simulink model "SIM_6DOF"  (R2021b)
settings: Solver=FixedStepAuto  StartTime=0.0  StopTime=D.Tfim  FixedStep=0.001  MaxStep=0.001  RelTol=1e-3
undefined symbols (not defined in the file or in its folder): c, D, dados, desv_emp, erro, F, Light, M, MIL, Newton, Raphson, wind
libraries: aerolibasang x7, sharedutil x3, aerolibwind2 x3, shared6dof x2, aerolibanim x1, aerolibatmos2 x1, simulink x1, dspmtrx3 x1, sharedtransform x1
settings Model: Creator=carlberto-old  LastModifiedBy=user
settings SolverCC: AlgebraicLoopSolver=LineSearch
settings DataIOCC: SaveFormat=Array  ReturnWorkspaceOutputs=off
settings DebuggingCC: SFMachineParentedDataDiag=warning  ArithmeticOperatorsInVariantConditions=warning
settings SFSimCC: SimUseLocalCustomCode=off  CustomCodeUndefinedFunction=UseInterfaceOnly
settings RTWCC: RTWUseLocalCustomCode=off

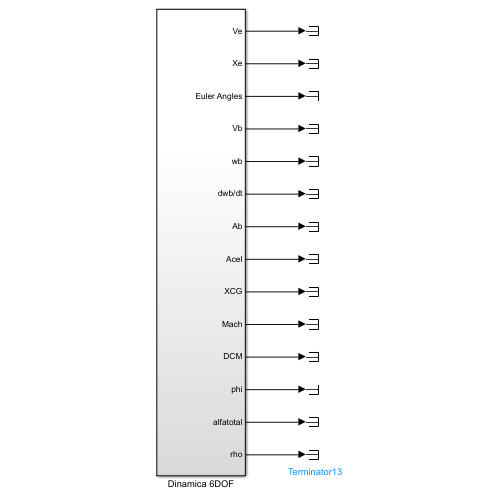
[thumbnail: Simulink's stored preview of the top-level diagram]
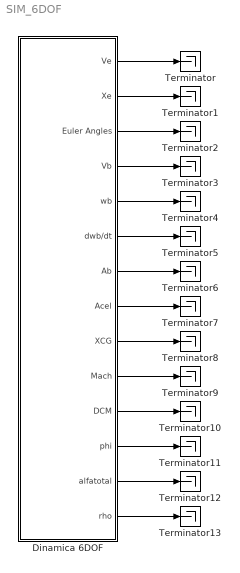
== system SIM_6DOF ==
  Dinamica 6DOF : Subsystem
  Terminator{,1..13} (14 alike) : Terminator
  wires:
  Dinamica 6DOF/3(Euler Angles) -> Terminator2/1
  Dinamica 6DOF/5(wb) -> Terminator4/1
  Dinamica 6DOF/1(Ve) -> Terminator/1
  Dinamica 6DOF/7(Ab) -> Terminator6/1
  Dinamica 6DOF/6(dwb/dt) -> Terminator5/1
  Dinamica 6DOF/11(DCM) -> Terminator10/1
  Dinamica 6DOF/9(XCG) -> Terminator8/1
  Dinamica 6DOF/8(Acel) -> Terminator7/1
  Dinamica 6DOF/10(Mach) -> Terminator9/1
  Dinamica 6DOF/12(phi) -> Terminator11/1
  Dinamica 6DOF/13(alfatotal) -> Terminator12/1
  Dinamica 6DOF/14(rho) -> Terminator13/1
  Dinamica 6DOF/2(Xe) -> Terminator1/1
  Dinamica 6DOF/4(Vb) -> Terminator3/1

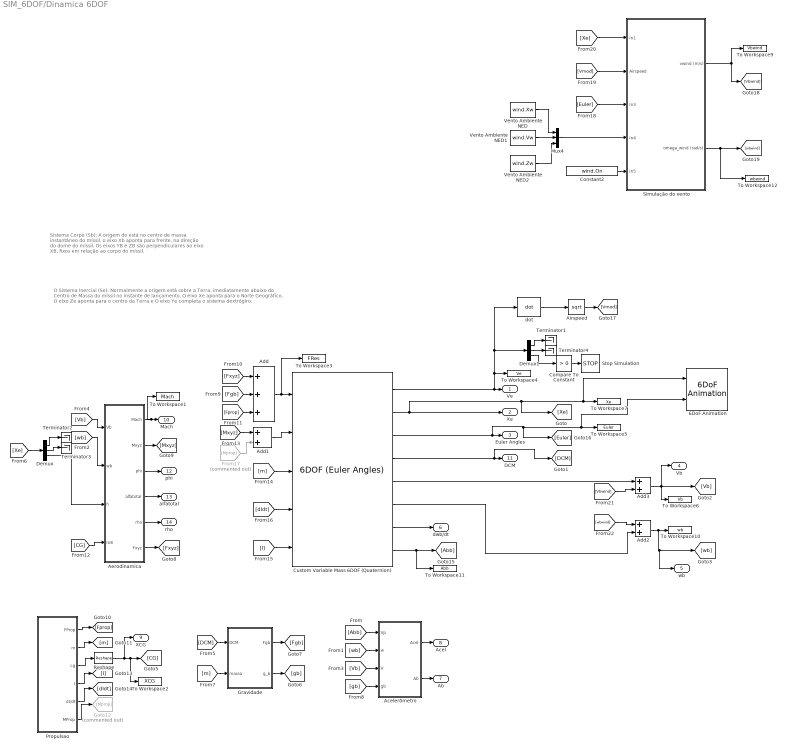
== system SIM_6DOF/Dinamica 6DOF ==
  note: O Sistema Inercial (Se):
      | Normalmente a origem está sobre a Terra, imediatamente abaixo do Centro de Massa do míssil no instante de lançamento.
      | O eixo Xe aponta para o Norte Geográfico,
      | O eixo Ze aponta para o centro da Terra e
      | O eixo Ye completa o sistema dextrógiro.
  note: Sistema Corpo (Sb):
      | A origem do está no centro de massa instantâneo do míssil.
      | o eixo Xb aponta para frente, na direção do dome do míssil.
      | Os eixos YB e ZB são perpendiculares ao eixo XB, fixos
      | em relação ao corpo do míssil.
  6DoF Animation : aerolibanim/6DoF Animation  u1=[0 4000 -2000 2000 -1000 6000]  u2=0.1  u3=1  u4=[0 0 0]  u5=Fly alongside  u6=[0 30 0]  u7=10  u8=on
  Acelerômetro : Subsystem
  Add : Sum  Inputs=+++
  Add1 : Sum
  Add2 : Sum
  Add3 : Sum
  Aerodinamica : Subsystem
  Airspeed : Sqrt  AlgorithmType=Newton-Raphson  SaturateOnIntegerOverflow=on
  Compare To Constant : simulink/Logic and Bit Operations/Compare To Constant  relop=>  const=0  OutDataTypeStr=boolean
  Constant2 : Constant  Value=wind.On
  Custom Variable Mass 6DOF (Quaternion) : shared6dof/6DOF (Euler Angles)  units=Metric (MKS)  mtype=Custom Variable  rep=Quaternion  xme_0=[0 0 -D.Alt0]  Vm_0=[D.U 0 0]  eul_0="[D.phi0  D.theta0   D.psi0]"  pm_0=[D.p0 D.q0 D.r0]  mass_0=1.0  mass_e=0.5  mass_f=2.0  inertia=eye(3)  inertia_e=eye(3)  inertia_f=2*eye(3)  k_quat=D.Kq  vre_flag=off  abi_flag=off  aMode=aMode  xme_statename=''  Vm_statename=''  eul_statename=''  quat_statename=''  pm_statename=''  mass_statename=''
      settings: SourceProductBaseCode=AE,PW,DR,MT,UV,VE
  Demux : Demux  Outputs=3
  Demux1 : Demux  Outputs=3
  From17 : From  Commented=on  GotoTag=Mprop
  Goto12 : Goto  Commented=on  GotoTag=Mprop
  Gravidade : Subsystem
  Mux4 : Mux  Inputs=3
  Propulsao : Subsystem
  Reshape : Reshape
  Simulação do vento : Subsystem
  Stop Simulation : Stop
  Terminator{1..4} (4 alike) : Terminator
  To Workspace1 : ToWorkspace  VariableName=Mach  SaveFormat=Timeseries  SampleTime=-1
  To Workspace10 : ToWorkspace  VariableName=wb  SaveFormat=Timeseries  SampleTime=-1
  To Workspace11 : ToWorkspace  VariableName=Abb  SaveFormat=Timeseries  SampleTime=-1
  To Workspace12 : ToWorkspace  VariableName=wbwind  SaveFormat=Timeseries  SampleTime=-1
  To Workspace2 : ToWorkspace  VariableName=XCG  SaveFormat=Timeseries  SampleTime=-1
  To Workspace3 : ToWorkspace  VariableName=FRes  SaveFormat=Timeseries  SampleTime=-1
  To Workspace4 : ToWorkspace  VariableName=Ve  SaveFormat=Timeseries  SampleTime=-1
  To Workspace5 : ToWorkspace  VariableName=Euler  SaveFormat=Timeseries  SampleTime=-1
  To Workspace6 : ToWorkspace  VariableName=Vb  SaveFormat=Timeseries  SampleTime=-1
  To Workspace7 : ToWorkspace  VariableName=Xe  SaveFormat=Timeseries  SampleTime=-1
  To Workspace9 : ToWorkspace  VariableName=Vbwind  SaveFormat=Timeseries  SampleTime=-1
  Vento Ambiente NED : Constant  Value=wind.Xw
  Vento Ambiente NED1 : Constant  Value=wind.Vw
  Vento Ambiente NED2 : Constant  Value=wind.Zw
  dot : aerolibasang/Incidence, Sideslip, & Airspeed/dot  SystemSampleTime=-1  VariantActivationTime=update diagram  Latency=0  AutoFrameSizeCalculation=off
      settings: SourceProductBaseCode=AE
  Ve : Outport  VectorParamsAs1DForOutWhenUnconnected=off
  Xe : Outport  Port=2  VectorParamsAs1DForOutWhenUnconnected=off
  Euler Angles : Outport  Port=3  VectorParamsAs1DForOutWhenUnconnected=off
  Vb : Outport  Port=4  VectorParamsAs1DForOutWhenUnconnected=off
  wb : Outport  Port=5  VectorParamsAs1DForOutWhenUnconnected=off
  dwb/dt : Outport  Port=6  VectorParamsAs1DForOutWhenUnconnected=off
  Ab : Outport  Port=7  VectorParamsAs1DForOutWhenUnconnected=off
  Acel : Outport  Port=8  VectorParamsAs1DForOutWhenUnconnected=off
  XCG : Outport  Port=9  VectorParamsAs1DForOutWhenUnconnected=off
  Mach : Outport  Port=10  VectorParamsAs1DForOutWhenUnconnected=off
  DCM : Outport  Port=11  VectorParamsAs1DForOutWhenUnconnected=off
  phi : Outport  Port=12  VectorParamsAs1DForOutWhenUnconnected=off
  alfatotal : Outport  Port=13  VectorParamsAs1DForOutWhenUnconnected=off
  rho : Outport  Port=14  VectorParamsAs1DForOutWhenUnconnected=off
  wires:
  Custom Variable Mass 6DOF (Quaternion)/1 -> To Workspace4/1, dot/1, Demux1/1, Ve/1
  Custom Variable Mass 6DOF (Quaternion)/7 -> dwb/dt/1
  Demux/1 -> Terminator2/1
  Demux/2 -> Terminator3/1
  Add/1 -> To Workspace3/1, Custom Variable Mass 6DOF (Quaternion)/1
  Custom Variable Mass 6DOF (Quaternion)/4 -> [DCM], DCM/1
  Demux/3 -> Aerodinamica/3(h)
  Aerodinamica/1(Mach) -> To Workspace1/1, Mach/1
  Propulsao/3(cg) -> Reshape/1
  [Abb] -> Acelerômetro/1(Vp)
  [wb] -> Acelerômetro/2(w)
  [wb] -> Aerodinamica/2(wb)
  [Vb] -> Acelerômetro/3(V)
  [Vb] -> Aerodinamica/1(Vb)
  [DCM] -> Gravidade/1(DCM)
  [Xe] -> Demux/1
  Acelerômetro/2(Ab) -> Ab/1
  [gb] -> Acelerômetro/4(gb)
  Aerodinamica/6(" Fxyz") -> [Fxyz]
  Aerodinamica/2(Mxyz) -> [Mxyz]
  Propulsao/1(FProp) -> [Fprop]
  Propulsao/2(m) -> [m]
  Propulsao/4(I) -> [I]
  Propulsao/5(dI/dt) -> [dIdt]
  [m] -> Custom Variable Mass 6DOF (Quaternion)/3
  [I] -> Custom Variable Mass 6DOF (Quaternion)/5
  [dIdt] -> Custom Variable Mass 6DOF (Quaternion)/4
  Custom Variable Mass 6DOF (Quaternion)/8 -> [Abb], To Workspace11/1
  Aerodinamica/3(phi) -> phi/1
  Aerodinamica/4(alfatotal) -> alfatotal/1
  Aerodinamica/5(rho) -> rho/1
  [m] -> Gravidade/2(massa)
  Gravidade/1(Fgb) -> [Fgb]
  Acelerômetro/1(Acel) -> Acel/1
  Gravidade/2(g_b) -> [gb]
  [Fprop] -> Add/3
  Add1/1 -> Custom Variable Mass 6DOF (Quaternion)/2
  Propulsao/6(MProp) -> Goto12/1
  Demux1/3 -> Compare To Constant/1
  Demux1/2 -> Terminator4/1
  Demux1/1 -> Terminator1/1
  Compare To Constant/1 -> Stop Simulation/1
  From17/1 -> Add1/2
  [Mxyz] -> Add1/1
  [Fgb] -> Add/2
  [Fxyz] -> Add/1
  [CG] -> Aerodinamica/4(In8)
  Custom Variable Mass 6DOF (Quaternion)/3 -> [Euler], 6DoF Animation/2, To Workspace5/1, Euler Angles/1
  Add3/1 -> Vb/1, To Workspace6/1, [Vb]
  Add2/1 -> wb/1, [wb], To Workspace10/1
  Custom Variable Mass 6DOF (Quaternion)/6 -> Add2/2
  Custom Variable Mass 6DOF (Quaternion)/5 -> Add3/1
  [Vbwind] -> Add3/2
  [wbwind] -> Add2/1
  Vento Ambiente NED2/1 -> Mux4/3
  Vento Ambiente NED1/1 -> Mux4/2
  Vento Ambiente NED/1 -> Mux4/1
  dot/1 -> Airspeed/1
  Airspeed/1 -> [Vmod]
  Custom Variable Mass 6DOF (Quaternion)/2 -> [Xe], 6DoF Animation/1, To Workspace7/1, Xe/1
  Reshape/1 -> XCG/1, To Workspace2/1, [CG]
  Simulação do vento/2(omega_wind (rad/s)) -> To Workspace12/1, [wbwind]
  Simulação do vento/1(vwind (m/s)) -> To Workspace9/1, [Vbwind]
  [Xe] -> Simulação do vento/1(In1)
  [Vmod] -> Simulação do vento/2(Airspeed)
  [Euler] -> Simulação do vento/3(In3)
  Mux4/1 -> Simulação do vento/4(In4)
  Constant2/1 -> Simulação do vento/5(In5)

== system SIM_6DOF/Dinamica 6DOF/Acelerômetro ==
  Vp : Inport
  w : Inport  Port=2
  V : Inport  Port=3
  gb : Inport  Port=4
  Add1 : Sum
  Add2 : Sum  Inputs=+-
  To Workspace4 : ToWorkspace  VariableName=Acel  SaveFormat=Timeseries  SampleTime=-1
  To Workspace5 : ToWorkspace  VariableName=Ab  SaveFormat=Timeseries  SampleTime=-1
  w x V : sharedutil/3x3 Cross Product  aMode=aMode
      settings: SourceProductBaseCode=AE,PW,DR,MT,UV,VE
  Acel : Outport  VectorParamsAs1DForOutWhenUnconnected=off
  Ab : Outport  Port=2  VectorParamsAs1DForOutWhenUnconnected=off
  wires:
  V/1 -> w x V/2
  w/1 -> w x V/1
  Add1/1 -> Add2/1, Ab/1, To Workspace5/1
  Add2/1 -> To Workspace4/1, Acel/1
  gb/1 -> Add2/2
  w x V/1 -> Add1/2
  Vp/1 -> Add1/1

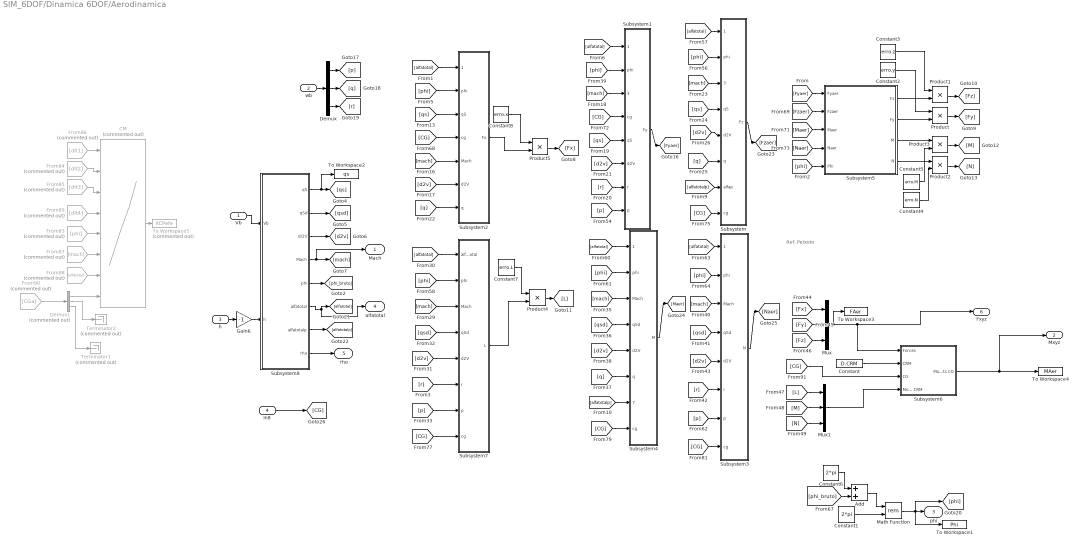
== system SIM_6DOF/Dinamica 6DOF/Aerodinamica ==
  note: Ref. Peixoto
  Vb : Inport
  wb : Inport  Port=2
  h : Inport  Port=3
  In8 : Inport  Port=4
  Add : Sum
  CM : Lookup_n-D  Commented=on  NumberOfTableDimensions=8  BreakpointsForDimension1=dados.delta1  BreakpointsForDimension2=dados.delta2  BreakpointsForDimension3=dados.delta3  BreakpointsForDimension4=dados.delta4  BreakpointsForDimension5=dados.phif  BreakpointsForDimension6=dados.mach  BreakpointsForDimension7=dados.alpha  BreakpointsForDimension8=dados.cg  Table=M.XCP  ExtrapMethod=Clip  InternalRulePriority=Speed  RndMeth=Simplest  InputSameDT=on
      settings: InputPortMap=u0,u1,u2,u3,u4,u5,u6,u7
  Constant : Constant  Value=D.CRM
  Constant1 : Constant  Value=2*pi
  Constant2 : Constant  Value=erro.y
  Constant3 : Constant  Value=erro.z
  Constant4 : Constant  Value=erro.N
  Constant5 : Constant  Value=erro.M
  Constant6 : Constant  Value=2*pi
  Constant7 : Constant  Value=erro.L
  Constant8 : Constant  Value=erro.x
  Demux : Demux  Outputs=3
  Demux1 : Demux  Commented=on  Outputs=3
  From83 : From  Commented=on  GotoTag=phi
  From84 : From  Commented=on  GotoTag=dlt2
  From85 : From  Commented=on  GotoTag=dlt3
  From86 : From  Commented=on  GotoTag=dlt1
  From87 : From  Commented=on  GotoTag=mach
  From88 : From  Commented=on  GotoTag=alfatotal
  From89 : From  Commented=on  GotoTag=dlt4
  From90 : From  Commented=on  GotoTag=CGa
  Gain6 : Gain  Gain=-1
  Math Function : Math  Operator=rem  SignedPower=on  SaturateOnIntegerOverflow=on
  Mux : Mux  Inputs=3
  Mux1 : Mux  Inputs=3
  Product{,1..5} (6 alike) : Product
  Subsystem : Subsystem
  Subsystem1 : Subsystem
  Subsystem2 : Subsystem
  Subsystem3 : Subsystem
  Subsystem4 : Subsystem
  Subsystem5 : Subsystem
  Subsystem6 : Subsystem
  Subsystem7 : Subsystem
  Subsystem8 : Subsystem
  Terminator1 : Terminator  Commented=on
  Terminator2 : Terminator  Commented=on
  To Workspace1 : ToWorkspace  VariableName=Phi  SaveFormat=Timeseries  SampleTime=-1
  To Workspace2 : ToWorkspace  VariableName=qs  SaveFormat=Timeseries  SampleTime=-1
  To Workspace3 : ToWorkspace  VariableName=FAer  SaveFormat=Timeseries  SampleTime=-1
  To Workspace4 : ToWorkspace  VariableName=MAer  SaveFormat=Timeseries  SampleTime=-1
  To Workspace5 : ToWorkspace  Commented=on  VariableName=XCPefe  SaveFormat=Timeseries  SampleTime=-1
  Mach : Outport  VectorParamsAs1DForOutWhenUnconnected=off
  Mxyz : Outport  Port=2  VectorParamsAs1DForOutWhenUnconnected=off
  phi : Outport  Port=3  VectorParamsAs1DForOutWhenUnconnected=off
  alfatotal : Outport  Port=4  VectorParamsAs1DForOutWhenUnconnected=off
  rho : Outport  Port=5  VectorParamsAs1DForOutWhenUnconnected=off
  " Fxyz" : Outport  Port=6  VectorParamsAs1DForOutWhenUnconnected=off
  wires:
  h/1 -> Gain6/1
  Mux/1 -> To Workspace3/1, Subsystem6/1(Forces), " Fxyz"/1
  wb/1 -> Demux/1
  Vb/1 -> Subsystem8/1(Vb)
  Gain6/1 -> Subsystem8/2(h)
  Constant/1 -> Subsystem6/2(CRM)
  [alfatotal] -> Subsystem2/1(alfatotal)
  [phi] -> Subsystem2/2(phi)
  [alfatotalp] -> Subsystem4/7(alfaponto)
  Subsystem8/1(qS) -> To Workspace2/1, [qs]
  Subsystem8/2(qSd) -> [qsd]
  Subsystem8/3(d/2V) -> [d2v]
  Subsystem8/4(Mach) -> Mach/1, [mach]
  [qs] -> Subsystem2/3(qS)
  [mach] -> Subsystem2/5("Mach ")
  [mach] -> Subsystem1/3("Mach ")
  [d2v] -> Subsystem7/5(d2V)
  [qsd] -> Subsystem7/4(qSd)
  [p] -> Subsystem7/7(p)
  [mach] -> Subsystem4/3("Mach ")
  [qsd] -> Subsystem4/4(qSd)
  [q] -> Subsystem4/6(q)
  [d2v] -> Subsystem4/5(d2V)
  [mach] -> Subsystem3/3("Mach ")
  [qsd] -> Subsystem3/4(qSd)
  [r] -> Subsystem3/6(r)
  [d2v] -> Subsystem3/5(d2V)
  [Fx] -> Mux/1
  [Fy] -> Mux/2
  [Fz] -> Mux/3
  [L] -> Mux1/1
  [M] -> Mux1/2
  [N] -> Mux1/3
  Subsystem8/6(alfatotal) -> [alfatotal], alfatotal/1
  [d2v] -> Subsystem2/6(d2V)
  [q] -> Subsystem2/7(q)
  [alfatotal] -> Subsystem1/1(alfatotal)
  [r] -> Subsystem1/7(r)
  [d2v] -> Subsystem1/6(d2V)
  [qs] -> Subsystem1/5(qS)
  [phi] -> Subsystem1/2(phi)
  [p] -> Subsystem1/8(p)
  [q] -> Subsystem/6(q)
  [mach] -> Subsystem/3("Mach ")
  [qs] -> Subsystem/4(qS)
  [d2v] -> Subsystem/5(d2V)
  [alfatotalp] -> Subsystem/7(alfap)
  [alfatotal] -> Subsystem/1(alfatotal)
  [phi] -> Subsystem/2(phi)
  [r] -> Subsystem7/6(r)
  [mach] -> Subsystem7/3("Mach ")
  [phi] -> Subsystem7/2(phi)
  [alfatotal] -> Subsystem7/1(alfatotal)
  [alfatotal] -> Subsystem4/1(alfatotal)
  [phi] -> Subsystem4/2(phi)
  [p] -> Subsystem3/7(p)
  [alfatotal] -> Subsystem3/1(alfatotal)
  [phi] -> Subsystem3/2(phi)
  Constant1/1 -> Math Function/2
  Demux/3 -> [r]
  Math Function/1 -> To Workspace1/1, [phi], phi/1
  Add/1 -> Math Function/1
  [phi] -> Subsystem5/5(Phi)
  [Fzaer] -> Subsystem5/2(Fzaer)
  [Fyaer] -> Subsystem5/1(Fyaer)
  [Maer] -> Subsystem5/3(Maer)
  [Naer] -> Subsystem5/4(Naer)
  Subsystem8/8(rho) -> rho/1
  Demux/1 -> [p]
  Constant6/1 -> Add/1
  Demux/2 -> [q]
  Subsystem8/7(alfatotalp) -> [alfatotalp]
  Subsystem4/1(M) -> [Maer]
  Subsystem8/5(phi) -> [phi_bruto]
  [phi_bruto] -> Add/2
  Subsystem3/1(N) -> [Naer]
  Subsystem/1(Fz) -> [Fzaer]
  Subsystem1/1(Fy) -> [Fyaer]
  Product/1 -> [Fy]
  Subsystem5/2(Fy) -> Product/2
  Constant2/1 -> Product/1
  Product1/1 -> [Fz]
  Constant3/1 -> Product1/1
  Subsystem5/1(Fz) -> Product1/2
  Product3/1 -> [M]
  Product2/1 -> [N]
  Subsystem5/3(M) -> Product3/1
  Subsystem5/4(N) -> Product2/1
  Constant5/1 -> Product3/2
  Constant4/1 -> Product2/2
  Subsystem2/1(Fx) -> Product5/2
  Product5/1 -> [Fx]
  Constant8/1 -> Product5/1
  Product4/1 -> [L]
  Subsystem7/1(L) -> Product4/2
  Constant7/1 -> Product4/1
  [CG] -> Subsystem2/4(cg)
  [CG] -> Subsystem1/4(cg)
  [CG] -> Subsystem/8(cg)
  [CG] -> Subsystem7/8(cg)
  [CG] -> Subsystem4/8(cg)
  [CG] -> Subsystem3/8(cg)
  From87/1 -> CM/6
  From86/1 -> CM/1
  From88/1 -> CM/7
  CM/1 -> To Workspace5/1
  From83/1 -> CM/5
  From89/1 -> CM/4
  From85/1 -> CM/3
  From84/1 -> CM/2
  In8/1 -> [CG]
  From90/1 -> Demux1/1
  Demux1/1 -> CM/8
  Demux1/2 -> Terminator2/1
  Demux1/3 -> Terminator1/1
  Subsystem6/1(Moments CG) -> Mxyz/1, To Workspace4/1
  [CG] -> Subsystem6/3(CG)
  Mux1/1 -> Subsystem6/4(Moments CRM)

== system SIM_6DOF/Dinamica 6DOF/Gravidade ==
  DCM : Inport
  massa : Inport  Port=2
  Constant2 : Constant  Value=0
  Constant3 : Constant  Value=0
  Constant4 : Constant  Value=c.g
  Mux : Mux  Inputs=3
  Product : Product
  "transform to Inertial axes " : shared6dof/6DOF (Euler Angles)/transform to Inertial axes   SystemSampleTime=-1  VariantActivationTime=update diagram  Latency=0  AutoFrameSizeCalculation=off
      settings: SourceProductBaseCode=AE,PW,DR,MT,UV,VE
  Fgb : Outport  VectorParamsAs1DForOutWhenUnconnected=off
  g_b : Outport  Port=2  VectorParamsAs1DForOutWhenUnconnected=off
  wires:
  Constant3/1 -> Mux/2
  Constant2/1 -> Mux/1
  Constant4/1 -> Mux/3
  Mux/1 -> g_b/1, Product/1
  DCM/1 -> "transform to Inertial axes "/2
  "transform to Inertial axes "/1 -> Fgb/1
  Product/1 -> "transform to Inertial axes "/1
  massa/1 -> Product/2

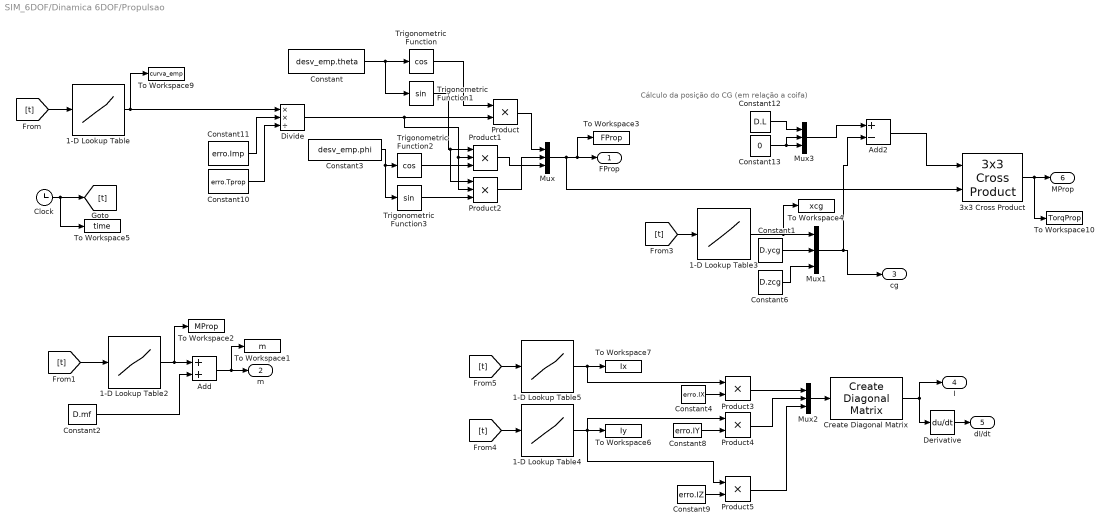
== system SIM_6DOF/Dinamica 6DOF/Propulsao ==
  note: Cálculo da posição do CG (em relação a coifa)
  1-D Lookup Table : Lookup_n-D  NumberOfTableDimensions=1  BreakpointsForDimension1=D.Empuxo(:,1)  Table=D.Empuxo(:,2)  ExtrapMethod=Clip  InternalRulePriority=Speed  RndMeth=Simplest  InputSameDT=on
  1-D Lookup Table2 : Lookup_n-D  NumberOfTableDimensions=1  BreakpointsForDimension1="[0  D.Tprop]"  Table=[D.mprop 0]  ExtrapMethod=Clip  InternalRulePriority=Speed  RndMeth=Simplest  InputSameDT=on
  1-D Lookup Table3 : Lookup_n-D  NumberOfTableDimensions=1  BreakpointsForDimension1="[0  D.Tprop]"  Table=[D.xcg0 D.xcgf]  ExtrapMethod=Clip  InternalRulePriority=Speed  RndMeth=Simplest  InputSameDT=on
  1-D Lookup Table4 : Lookup_n-D  NumberOfTableDimensions=1  BreakpointsForDimension1=[0 D.Tprop/2 D.Tprop]  Table=[D.Iy0 D.Iym D.Iyf]  ExtrapMethod=Clip  InternalRulePriority=Speed  RndMeth=Simplest  InputSameDT=on
  1-D Lookup Table5 : Lookup_n-D  NumberOfTableDimensions=1  BreakpointsForDimension1=[0 D.Tprop/2 D.Tprop]  Table=[D.Ix0 D.Ixm D.Ixf]  ExtrapMethod=Clip  InternalRulePriority=Speed  RndMeth=Simplest  InputSameDT=on
  3x3 Cross Product : sharedutil/3x3 Cross Product  aMode=aMode
      settings: SourceProductBaseCode=AE,PW,DR,MT,UV,VE
  Add : Sum
  Add2 : Sum  Inputs=+-
  Clock : Clock
  Constant : Constant  Value=desv_emp.theta
  Constant1 : Constant  Value=D.ycg
  Constant10 : Constant  Value=erro.Tprop
  Constant11 : Constant  Value=erro.Imp
  Constant12 : Constant  Value=D.L
  Constant13 : Constant  Value=0
  Constant2 : Constant  Value=D.mf
  Constant3 : Constant  Value=desv_emp.phi
  Constant4 : Constant  Value=erro.IX
  Constant6 : Constant  Value=D.zcg
  Constant8 : Constant  Value=erro.IY
  Constant9 : Constant  Value=erro.IZ
  Create Diagonal Matrix : dspmtrx3/Create Diagonal Matrix
      settings: SourceProductBaseCode=DS
  Derivative : Derivative
  Divide : Product  Inputs=**/
  Mux{,1..3} (4 alike) : Mux  Inputs=3
  Product{,3..5} (4 alike) : Product
  Product1 : Product  Inputs=3
  Product2 : Product  Inputs=3
  To Workspace1 : ToWorkspace  VariableName=m  SaveFormat=Timeseries  SampleTime=-1
  To Workspace10 : ToWorkspace  VariableName=TorqProp  SaveFormat=Timeseries  SampleTime=-1
  To Workspace2 : ToWorkspace  VariableName=MProp  SaveFormat=Timeseries  SampleTime=-1
  To Workspace3 : ToWorkspace  VariableName=FProp  SaveFormat=Timeseries  SampleTime=-1
  To Workspace4 : ToWorkspace  VariableName=xcg  SaveFormat=Timeseries  SampleTime=-1
  To Workspace5 : ToWorkspace  VariableName=time  SaveFormat=Timeseries  SampleTime=-1
  To Workspace6 : ToWorkspace  VariableName=Iy  SaveFormat=Timeseries  SampleTime=-1
  To Workspace7 : ToWorkspace  VariableName=Ix  SaveFormat=Timeseries  SampleTime=-1
  To Workspace9 : ToWorkspace  VariableName=curva_emp  SaveFormat=Timeseries  SampleTime=-1
  Trigonometric Function : Trigonometry  Operator=cos
  Trigonometric Function1 : Trigonometry
  Trigonometric Function2 : Trigonometry  Operator=cos
  Trigonometric Function3 : Trigonometry
  FProp : Outport  VectorParamsAs1DForOutWhenUnconnected=off
  m : Outport  Port=2  VectorParamsAs1DForOutWhenUnconnected=off
  cg : Outport  Port=3  VectorParamsAs1DForOutWhenUnconnected=off
  I : Outport  Port=4  VectorParamsAs1DForOutWhenUnconnected=off
  dI/dt : Outport  Port=5  VectorParamsAs1DForOutWhenUnconnected=off
  MProp : Outport  Port=6  VectorParamsAs1DForOutWhenUnconnected=off
  wires:
  Mux/1 -> 3x3 Cross Product/2, FProp/1, To Workspace3/1
  1-D Lookup Table2/1 -> To Workspace2/1, Add/1
  Add/1 -> m/1, To Workspace1/1
  Constant2/1 -> Add/2
  Derivative/1 -> dI/dt/1
  1-D Lookup Table3/1 -> To Workspace4/1, Mux1/1
  Create Diagonal Matrix/1 -> I/1, Derivative/1
  1-D Lookup Table4/1 -> Product5/1, Product4/1, To Workspace6/1
  Mux2/1 -> Create Diagonal Matrix/1
  Clock/1 -> [t], To Workspace5/1
  [t] -> 1-D Lookup Table/1
  [t] -> 1-D Lookup Table2/1
  [t] -> 1-D Lookup Table3/1
  [t] -> 1-D Lookup Table5/1
  [t] -> 1-D Lookup Table4/1
  1-D Lookup Table5/1 -> Product3/1, To Workspace7/1
  Constant/1 -> Trigonometric Function1/1, Trigonometric Function/1
  Trigonometric Function/1 -> Product/1
  Product/1 -> Mux/1
  Constant3/1 -> Trigonometric Function3/1, Trigonometric Function2/1
  Trigonometric Function3/1 -> Product2/3
  Trigonometric Function2/1 -> Product1/3
  Trigonometric Function1/1 -> Product2/1, Product1/1
  Constant1/1 -> Mux1/2
  Constant6/1 -> Mux1/3
  3x3 Cross Product/1 -> To Workspace10/1, MProp/1
  Product3/1 -> Mux2/1
  Product5/1 -> Mux2/3
  Product4/1 -> Mux2/2
  Constant4/1 -> Product3/2
  Constant8/1 -> Product4/2
  Constant9/1 -> Product5/2
  Constant10/1 -> Divide/3
  Constant11/1 -> Divide/2
  1-D Lookup Table/1 -> To Workspace9/1, Divide/1
  Divide/1 -> Product2/2, Product1/2, Product/2
  Product2/1 -> Mux/2
  Product1/1 -> Mux/3
  Mux3/1 -> Add2/1
  Constant13/1 -> Mux3/3, Mux3/2
  Constant12/1 -> Mux3/1
  Mux1/1 -> cg/1, Add2/2
  Add2/1 -> 3x3 Cross Product/1

== system SIM_6DOF/Dinamica 6DOF/Simulação do vento ==
  In1 : Inport
  Airspeed : Inport  Port=2
  In3 : Inport  Port=3
  In4 : Inport  Port=4
  In5 : Inport  Port=5
  Constant1 : Constant  Value=0
  Demux2 : Demux  Outputs=3
  Discrete Wind Gust Model1 : aerolibwind2/Discrete Wind Gust Model  units=Metric (MKS)  Gx=on  Gy=on  Gz=on  t_0=5  d_m=[120 120 80]  v_m=[3.5 3.5 3.0]
  Dryden Wind Turbulence Model (Continuous (+q +r))1 : aerolibwind2/Dryden Wind Turbulence Model  (Continuous (+q -r))  units=Metric (MKS)  spec=MIL-F-8785C  model=Continuous Dryden (+q +r)  W20=15  Wdeg=0  TurbProb=10^-2 - Light  L_high=533.4  Wingspan=10  ts=0.1  Seed=[23341 23342 23343 23344]  T_on=on
  Multiport Switch : MultiPortSwitch  Inputs=4
  Mux{,1..3} (4 alike) : Mux  Inputs=[3 3]
  Product : Product  Multiplication=Matrix(*)
  Rotation Angles to Direction Cosine Matrix1 : sharedtransform/Rotation Angles to Direction Cosine Matrix  rotationOrder=ZYX  aMode=aMode
      settings: SourceProductBaseCode=AE,PW,DR,MT,UV,VE
  Selector : Selector  InputPortWidth=6  IndexOptions=Index vector (dialog)  Indices=[1 2 3]  OutputSizes=1
  Selector1 : Selector  InputPortWidth=6  IndexOptions=Index vector (dialog)  Indices=[4 5 6]  OutputSizes=1
  Sum : Sum  Inputs=|++  InputSameDT=on  SaturateOnIntegerOverflow=on  OutDataTypeStr=Inherit: Same as first input
  Sum1 : Sum  Inputs=|++  InputSameDT=on  SaturateOnIntegerOverflow=on  OutDataTypeStr=Inherit: Same as first input
  Sum2 : Sum  Inputs=|++  InputSameDT=on  SaturateOnIntegerOverflow=on  OutDataTypeStr=Inherit: Same as first input
  Sum3 : Sum  Inputs=+++  InputSameDT=on  SaturateOnIntegerOverflow=on  OutDataTypeStr=Inherit: Same as first input
  Switch : Switch  Threshold=1
  Terminator5 : Terminator
  Terminator6 : Terminator
  Wind Shear Model1 : aerolibwind2/Wind Shear Model  units=Metric (MKS)  phase=Category C - Terminal Flight Phase  W_20=15  Wdeg=0
  Wind Velocity Components2 : Constant  Value=[0 0 0]
  Wind Velocity Components6 : Constant  Value=[0 0 0]
  tipo : Constant  Value=wind.tipo
  vwind (m/s) : Outport
  omega_wind (rad/s) : Outport  Port=2
  wires:
  In1/1 -> Demux2/1
  Product/1 -> Sum/2, Sum3/3, Sum2/2, Sum1/2
  Switch/1 -> Selector1/1, Selector/1
  Airspeed/1 -> Discrete Wind Gust Model1/1, Dryden Wind Turbulence Model (Continuous (+q +r))1/2
  Dryden Wind Turbulence Model (Continuous (+q +r))1/2 -> Mux3/2, Mux/2
  Wind Velocity Components6/1 -> Mux2/2
  Wind Shear Model1/1 -> Sum1/1
  Rotation Angles to Direction Cosine Matrix1/1 -> Dryden Wind Turbulence Model (Continuous (+q +r))1/3, Product/1, Wind Shear Model1/2
  Mux1/1 -> Multiport Switch/3
  Sum1/1 -> Mux1/1
  Dryden Wind Turbulence Model (Continuous (+q +r))1/1 -> Sum/1, Sum3/1
  Mux/1 -> Multiport Switch/2
  Sum/1 -> Mux/1
  Mux2/1 -> Multiport Switch/4
  In4/1 -> Product/2
  Sum2/1 -> Mux2/1
  tipo/1 -> Multiport Switch/1
  Constant1/1 -> Switch/3
  Mux3/1 -> Multiport Switch/5
  Wind Velocity Components2/1 -> Mux1/2
  Discrete Wind Gust Model1/1 -> Sum2/1, Sum3/2
  Multiport Switch/1 -> Switch/1
  Demux2/1 -> Terminator5/1
  Demux2/3 -> Wind Shear Model1/1, Dryden Wind Turbulence Model (Continuous (+q +r))1/1
  Sum3/1 -> Mux3/1
  Selector1/1 -> omega_wind (rad/s)/1  "omega_wind (rad/s)"
  Demux2/2 -> Terminator6/1
  Selector/1 -> vwind (m/s)/1  "vwind (m/s)"
  In3/1 -> Rotation Angles to Direction Cosine Matrix1/1
  In5/1 -> Switch/2

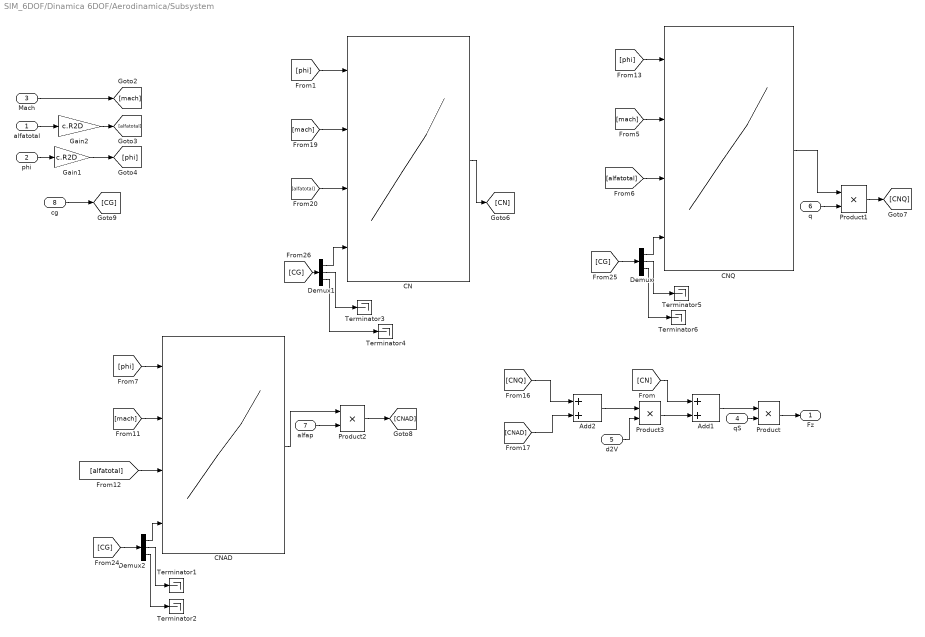
== system SIM_6DOF/Dinamica 6DOF/Aerodinamica/Subsystem ==
  alfatotal : Inport
  phi : Inport  Port=2
  "Mach " : Inport  Port=3
  qS : Inport  Port=4
  d2V : Inport  Port=5
  q : Inport  Port=6
  alfap : Inport  Port=7
  cg : Inport  Port=8
  Add1 : Sum
  Add2 : Sum
  CN : Lookup_n-D  NumberOfTableDimensions=4  BreakpointsForDimension1=dados.phif  BreakpointsForDimension2=dados.mach  BreakpointsForDimension3=dados.alpha  BreakpointsForDimension4=dados.cg  BreakpointsForDimension5=dados.phif  BreakpointsForDimension6=dados.mach  BreakpointsForDimension7=dados.alpha  BreakpointsForDimension8=dados.cg  Table=M.CN  ExtrapMethod=Clip  InternalRulePriority=Speed  RndMeth=Simplest  InputSameDT=on
      settings: InputPortMap=u0,u1,u2,u3
  CNAD : Lookup_n-D  NumberOfTableDimensions=4  BreakpointsForDimension1=dados.phif  BreakpointsForDimension2=dados.mach  BreakpointsForDimension3=dados.alpha  BreakpointsForDimension4=dados.cg  BreakpointsForDimension5=dados.phif  BreakpointsForDimension6=dados.mach  BreakpointsForDimension7=dados.alpha  BreakpointsForDimension8=dados.cg  Table=M.CNAD  ExtrapMethod=Clip  InternalRulePriority=Speed  RndMeth=Simplest  InputSameDT=on
      settings: InputPortMap=u0,u1,u2,u3
  CNQ : Lookup_n-D  NumberOfTableDimensions=4  BreakpointsForDimension1=dados.phif  BreakpointsForDimension2=dados.mach  BreakpointsForDimension3=dados.alpha  BreakpointsForDimension4=dados.cg  BreakpointsForDimension5=dados.phif  BreakpointsForDimension6=dados.mach  BreakpointsForDimension7=dados.alpha  BreakpointsForDimension8=dados.cg  Table=M.CNQ  ExtrapMethod=Clip  InternalRulePriority=Speed  RndMeth=Simplest  InputSameDT=on
      settings: InputPortMap=u0,u1,u2,u3
  Demux : Demux  Outputs=3
  Demux1 : Demux  Outputs=3
  Demux2 : Demux  Outputs=3
  Gain1 : Gain  Gain=c.R2D
  Gain2 : Gain  Gain=c.R2D
  Product{,1..3} (4 alike) : Product
  Terminator{1..6} (6 alike) : Terminator
  Fz : Outport  VectorParamsAs1DForOutWhenUnconnected=off
  wires:
  Add1/1 -> Product/1
  phi/1 -> Gain1/1
  Gain2/1 -> [alfatotal]
  "Mach "/1 -> [mach]
  Gain1/1 -> [phi]
  alfatotal/1 -> Gain2/1
  q/1 -> Product1/2
  CNQ/1 -> Product1/1
  qS/1 -> Product/2
  alfap/1 -> Product2/2
  CNAD/1 -> Product2/1
  Add2/1 -> Product3/1
  d2V/1 -> Product3/2
  Product/1 -> Fz/1
  Product3/1 -> Add1/2
  CN/1 -> [CN]
  Product1/1 -> [CNQ]
  Product2/1 -> [CNAD]
  [CN] -> Add1/1
  [CNQ] -> Add2/1
  [CNAD] -> Add2/2
  cg/1 -> [CG]
  [alfatotal] -> CNAD/3
  [mach] -> CNAD/2
  [phi] -> CNAD/1
  [alfatotal] -> CNQ/3
  [mach] -> CNQ/2
  [phi] -> CNQ/1
  [alfatotal] -> CN/3
  [mach] -> CN/2
  [phi] -> CN/1
  [CG] -> Demux/1
  Demux/1 -> CNQ/4
  [CG] -> Demux1/1
  Demux1/1 -> CN/4
  Demux2/1 -> CNAD/4
  [CG] -> Demux2/1
  Demux2/2 -> Terminator1/1
  Demux2/3 -> Terminator2/1
  Demux1/2 -> Terminator3/1
  Demux1/3 -> Terminator4/1
  Demux/2 -> Terminator5/1
  Demux/3 -> Terminator6/1

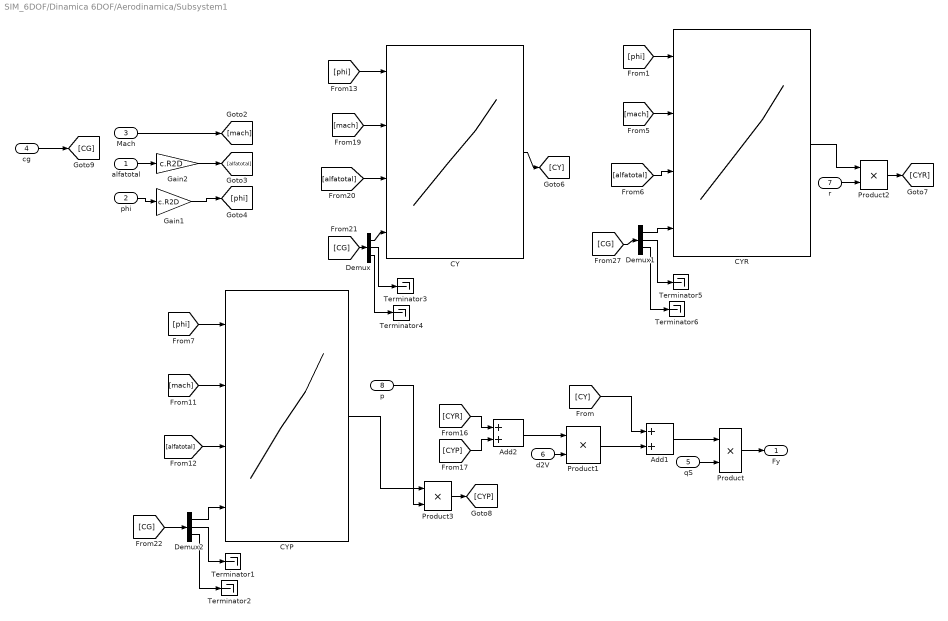
== system SIM_6DOF/Dinamica 6DOF/Aerodinamica/Subsystem1 ==
  alfatotal : Inport
  phi : Inport  Port=2
  "Mach " : Inport  Port=3
  cg : Inport  Port=4
  qS : Inport  Port=5
  d2V : Inport  Port=6
  r : Inport  Port=7
  p : Inport  Port=8
  Add1 : Sum
  Add2 : Sum
  CY : Lookup_n-D  NumberOfTableDimensions=4  BreakpointsForDimension1=dados.phif  BreakpointsForDimension2=dados.mach  BreakpointsForDimension3=dados.alpha  BreakpointsForDimension4=dados.cg  BreakpointsForDimension5=dados.phif  BreakpointsForDimension6=dados.mach  BreakpointsForDimension7=dados.alpha  BreakpointsForDimension8=dados.cg  Table=M.CY  ExtrapMethod=Clip  InternalRulePriority=Speed  RndMeth=Simplest  InputSameDT=on
      settings: InputPortMap=u0,u1,u2,u3
  CYP : Lookup_n-D  NumberOfTableDimensions=4  BreakpointsForDimension1=dados.phif  BreakpointsForDimension2=dados.mach  BreakpointsForDimension3=dados.alpha  BreakpointsForDimension4=dados.cg  BreakpointsForDimension5=dados.phif  BreakpointsForDimension6=dados.mach  BreakpointsForDimension7=dados.alpha  BreakpointsForDimension8=dados.cg  Table=M.CYP  ExtrapMethod=Clip  InternalRulePriority=Speed  RndMeth=Simplest  InputSameDT=on
      settings: InputPortMap=u0,u1,u2,u3
  CYR : Lookup_n-D  NumberOfTableDimensions=4  BreakpointsForDimension1=dados.phif  BreakpointsForDimension2=dados.mach  BreakpointsForDimension3=dados.alpha  BreakpointsForDimension4=dados.cg  BreakpointsForDimension5=dados.phif  BreakpointsForDimension6=dados.mach  BreakpointsForDimension7=dados.alpha  BreakpointsForDimension8=dados.cg  Table=M.CYR  ExtrapMethod=Clip  InternalRulePriority=Speed  RndMeth=Simplest  InputSameDT=on
      settings: InputPortMap=u0,u1,u2,u3
  Demux : Demux  Outputs=3
  Demux1 : Demux  Outputs=3
  Demux2 : Demux  Outputs=3
  Gain1 : Gain  Gain=c.R2D
  Gain2 : Gain  Gain=c.R2D
  Product{,1..3} (4 alike) : Product
  Terminator{1..6} (6 alike) : Terminator
  Fy : Outport  VectorParamsAs1DForOutWhenUnconnected=off
  wires:
  Gain1/1 -> [phi]
  "Mach "/1 -> [mach]
  alfatotal/1 -> Gain2/1
  Gain2/1 -> [alfatotal]
  phi/1 -> Gain1/1
  Add1/1 -> Product/1
  qS/1 -> Product/2
  CYR/1 -> Product2/1
  r/1 -> Product2/2
  CYP/1 -> Product3/1
  p/1 -> Product3/2
  d2V/1 -> Product1/2
  Add2/1 -> Product1/1
  Product1/1 -> Add1/2
  Product/1 -> Fy/1
  [alfatotal] -> CY/3
  CY/1 -> [CY]
  Product2/1 -> [CYR]
  Product3/1 -> [CYP]
  [CY] -> Add1/1
  [CYR] -> Add2/1
  [CYP] -> Add2/2
  cg/1 -> [CG]
  [mach] -> CY/2
  [phi] -> CY/1
  Demux1/1 -> CYR/4
  [alfatotal] -> CYR/3
  [mach] -> CYR/2
  [phi] -> CYR/1
  Demux2/1 -> CYP/4
  [alfatotal] -> CYP/3
  [mach] -> CYP/2
  [phi] -> CYP/1
  Demux/1 -> CY/4
  [CG] -> Demux/1
  [CG] -> Demux1/1
  [CG] -> Demux2/1
  Demux2/2 -> Terminator1/1
  Demux2/3 -> Terminator2/1
  Demux/2 -> Terminator3/1
  Demux/3 -> Terminator4/1
  Demux1/2 -> Terminator5/1
  Demux1/3 -> Terminator6/1

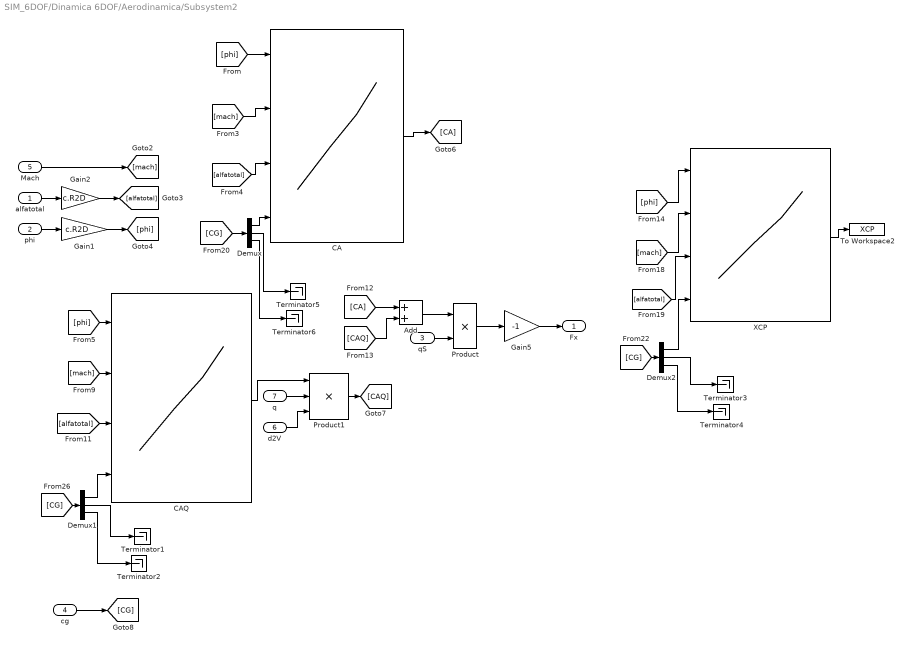
== system SIM_6DOF/Dinamica 6DOF/Aerodinamica/Subsystem2 ==
  alfatotal : Inport
  phi : Inport  Port=2
  qS : Inport  Port=3
  cg : Inport  Port=4
  "Mach " : Inport  Port=5
  d2V : Inport  Port=6
  q : Inport  Port=7
  Add : Sum
  CA : Lookup_n-D  NumberOfTableDimensions=4  BreakpointsForDimension1=dados.phif  BreakpointsForDimension2=dados.mach  BreakpointsForDimension3=dados.alpha  BreakpointsForDimension4=dados.cg  BreakpointsForDimension5=dados.phif  BreakpointsForDimension6=dados.mach  BreakpointsForDimension7=dados.alpha  BreakpointsForDimension8=dados.cg  Table=M.CA  ExtrapMethod=Clip  InternalRulePriority=Speed  RndMeth=Simplest  InputSameDT=on
      settings: InputPortMap=u0,u1,u2,u3
  CAQ : Lookup_n-D  NumberOfTableDimensions=4  BreakpointsForDimension1=dados.phif  BreakpointsForDimension2=dados.mach  BreakpointsForDimension3=dados.alpha  BreakpointsForDimension4=dados.cg  BreakpointsForDimension5=dados.phif  BreakpointsForDimension6=dados.mach  BreakpointsForDimension7=dados.alpha  BreakpointsForDimension8=dados.cg  Table=M.CAQ  ExtrapMethod=Clip  InternalRulePriority=Speed  RndMeth=Simplest  InputSameDT=on
      settings: InputPortMap=u0,u1,u2,u3
  Demux : Demux  Outputs=3
  Demux1 : Demux  Outputs=3
  Demux2 : Demux  Outputs=3
  Gain1 : Gain  Gain=c.R2D
  Gain2 : Gain  Gain=c.R2D
  Gain5 : Gain  Gain=-1
  Product : Product
  Product1 : Product  Inputs=3
  Terminator{1..6} (6 alike) : Terminator
  To Workspace2 : ToWorkspace  VariableName=XCP  SaveFormat=Timeseries  SampleTime=-1
  XCP : Lookup_n-D  NumberOfTableDimensions=4  BreakpointsForDimension1=dados.phif  BreakpointsForDimension2=dados.mach  BreakpointsForDimension3=dados.alpha  BreakpointsForDimension4=dados.cg  BreakpointsForDimension5=dados.phif  BreakpointsForDimension6=dados.mach  BreakpointsForDimension7=dados.alpha  BreakpointsForDimension8=dados.cg  Table=M.XCP  ExtrapMethod=Clip  InternalRulePriority=Speed  RndMeth=Simplest  InputSameDT=on
      settings: InputPortMap=u0,u1,u2,u3
  Fx : Outport  VectorParamsAs1DForOutWhenUnconnected=off
  wires:
  alfatotal/1 -> Gain2/1
  phi/1 -> Gain1/1
  Product/1 -> Gain5/1
  qS/1 -> Product/2
  Gain5/1 -> Fx/1
  "Mach "/1 -> [mach]
  Gain2/1 -> [alfatotal]
  Gain1/1 -> [phi]
  d2V/1 -> Product1/3
  CAQ/1 -> Product1/1
  q/1 -> Product1/2
  Add/1 -> Product/1
  [phi] -> CAQ/1
  CA/1 -> [CA]
  Product1/1 -> [CAQ]
  [CAQ] -> Add/2
  XCP/1 -> To Workspace2/1
  cg/1 -> [CG]
  [phi] -> CA/1
  [mach] -> CA/2
  [alfatotal] -> CA/3
  Demux1/1 -> CAQ/4
  [alfatotal] -> CAQ/3
  [mach] -> CAQ/2
  [phi] -> XCP/1
  [mach] -> XCP/2
  [alfatotal] -> XCP/3
  [CA] -> Add/1
  Demux/1 -> CA/4
  [CG] -> Demux/1
  [CG] -> Demux1/1
  [CG] -> Demux2/1
  Demux1/2 -> Terminator1/1
  Demux1/3 -> Terminator2/1
  Demux2/2 -> Terminator3/1
  Demux2/3 -> Terminator4/1
  Demux/2 -> Terminator5/1
  Demux/3 -> Terminator6/1
  Demux2/1 -> XCP/4

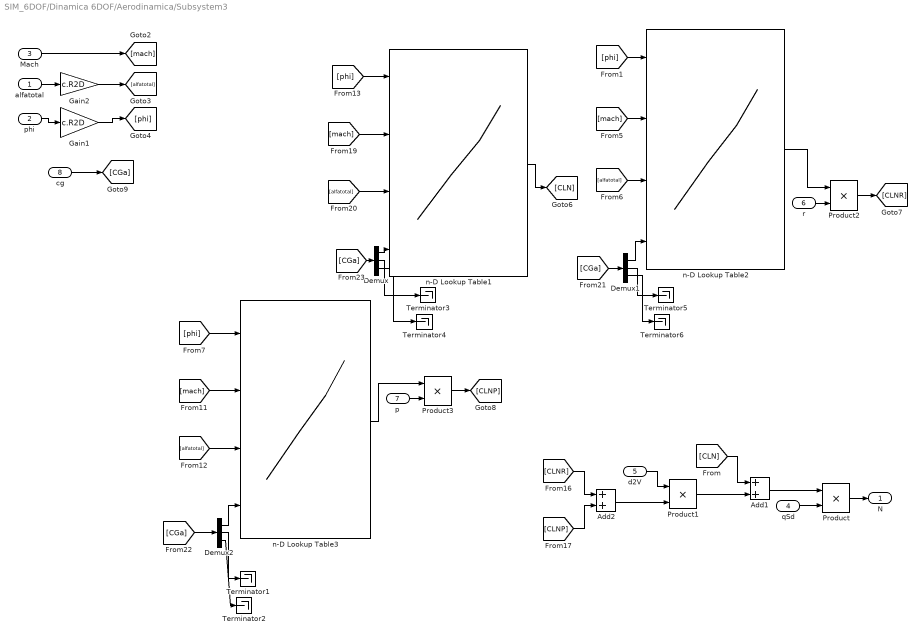
== system SIM_6DOF/Dinamica 6DOF/Aerodinamica/Subsystem3 ==
  alfatotal : Inport
  phi : Inport  Port=2
  "Mach " : Inport  Port=3
  qSd : Inport  Port=4
  d2V : Inport  Port=5
  r : Inport  Port=6
  p : Inport  Port=7
  cg : Inport  Port=8
  Add1 : Sum
  Add2 : Sum
  Demux : Demux  Outputs=3
  Demux1 : Demux  Outputs=3
  Demux2 : Demux  Outputs=3
  Gain1 : Gain  Gain=c.R2D
  Gain2 : Gain  Gain=c.R2D
  Product{,1..3} (4 alike) : Product
  Terminator{1..6} (6 alike) : Terminator
  n-D Lookup Table1 : Lookup_n-D  NumberOfTableDimensions=4  BreakpointsForDimension1=dados.phif  BreakpointsForDimension2=dados.mach  BreakpointsForDimension3=dados.alpha  BreakpointsForDimension4=dados.cg  BreakpointsForDimension5=dados.phif  BreakpointsForDimension6=dados.mach  BreakpointsForDimension7=dados.alpha  BreakpointsForDimension8=dados.cg  Table=M.CLN  ExtrapMethod=Clip  InternalRulePriority=Speed  RndMeth=Simplest  InputSameDT=on
      settings: InputPortMap=u0,u1,u2,u3
  n-D Lookup Table2 : Lookup_n-D  NumberOfTableDimensions=4  BreakpointsForDimension1=dados.phif  BreakpointsForDimension2=dados.mach  BreakpointsForDimension3=dados.alpha  BreakpointsForDimension4=dados.cg  BreakpointsForDimension5=dados.phif  BreakpointsForDimension6=dados.mach  BreakpointsForDimension7=dados.alpha  BreakpointsForDimension8=dados.cg  Table=M.CLNR  ExtrapMethod=Clip  InternalRulePriority=Speed  RndMeth=Simplest  InputSameDT=on
      settings: InputPortMap=u0,u1,u2,u3
  n-D Lookup Table3 : Lookup_n-D  NumberOfTableDimensions=4  BreakpointsForDimension1=dados.phif  BreakpointsForDimension2=dados.mach  BreakpointsForDimension3=dados.alpha  BreakpointsForDimension4=dados.cg  BreakpointsForDimension5=dados.phif  BreakpointsForDimension6=dados.mach  BreakpointsForDimension7=dados.alpha  BreakpointsForDimension8=dados.cg  Table=M.CLNP  ExtrapMethod=Clip  InternalRulePriority=Speed  RndMeth=Simplest  InputSameDT=on
      settings: InputPortMap=u0,u1,u2,u3
  N : Outport  VectorParamsAs1DForOutWhenUnconnected=off
  wires:
  phi/1 -> Gain1/1
  Gain2/1 -> [alfatotal]
  Add1/1 -> Product/1
  "Mach "/1 -> [mach]
  r/1 -> Product2/2
  n-D Lookup Table3/1 -> Product3/1
  qSd/1 -> Product/2
  alfatotal/1 -> Gain2/1
  Gain1/1 -> [phi]
  n-D Lookup Table2/1 -> Product2/1
  p/1 -> Product3/2
  Add2/1 -> Product1/2
  d2V/1 -> Product1/1
  Product1/1 -> Add1/2
  Product/1 -> N/1
  n-D Lookup Table1/1 -> [CLN]
  Product2/1 -> [CLNR]
  Product3/1 -> [CLNP]
  [CLN] -> Add1/1
  [CLNR] -> Add2/1
  [CLNP] -> Add2/2
  cg/1 -> [CGa]
  [alfatotal] -> n-D Lookup Table3/3
  [mach] -> n-D Lookup Table3/2
  [phi] -> n-D Lookup Table3/1
  [alfatotal] -> n-D Lookup Table2/3
  [mach] -> n-D Lookup Table2/2
  [phi] -> n-D Lookup Table2/1
  [alfatotal] -> n-D Lookup Table1/3
  [mach] -> n-D Lookup Table1/2
  [phi] -> n-D Lookup Table1/1
  [CGa] -> Demux/1
  Demux/1 -> n-D Lookup Table1/4
  [CGa] -> Demux1/1
  Demux1/1 -> n-D Lookup Table2/4
  Demux2/1 -> n-D Lookup Table3/4
  [CGa] -> Demux2/1
  Demux2/2 -> Terminator1/1
  Demux2/3 -> Terminator2/1
  Demux/2 -> Terminator3/1
  Demux/3 -> Terminator4/1
  Demux1/2 -> Terminator5/1
  Demux1/3 -> Terminator6/1

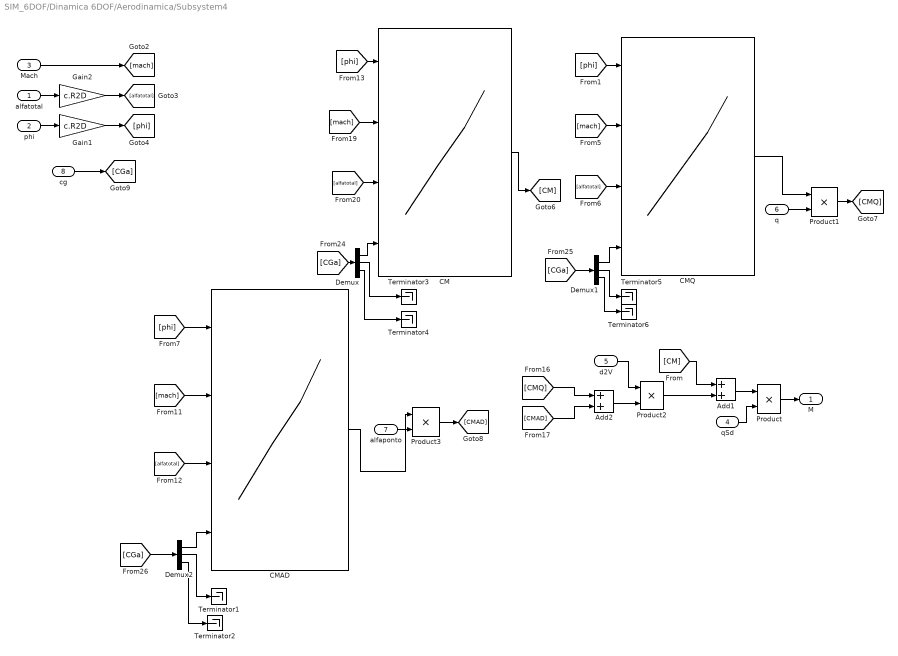
== system SIM_6DOF/Dinamica 6DOF/Aerodinamica/Subsystem4 ==
  alfatotal : Inport
  phi : Inport  Port=2
  "Mach " : Inport  Port=3
  qSd : Inport  Port=4
  d2V : Inport  Port=5
  q : Inport  Port=6
  alfaponto : Inport  Port=7
  cg : Inport  Port=8
  Add1 : Sum
  Add2 : Sum
  CM : Lookup_n-D  NumberOfTableDimensions=4  BreakpointsForDimension1=dados.phif  BreakpointsForDimension2=dados.mach  BreakpointsForDimension3=dados.alpha  BreakpointsForDimension4=dados.cg  BreakpointsForDimension5=dados.phif  BreakpointsForDimension6=dados.mach  BreakpointsForDimension7=dados.alpha  BreakpointsForDimension8=dados.cg  Table=M.CM  ExtrapMethod=Clip  InternalRulePriority=Speed  RndMeth=Simplest  InputSameDT=on
      settings: InputPortMap=u0,u1,u2,u3
  CMAD : Lookup_n-D  NumberOfTableDimensions=4  BreakpointsForDimension1=dados.phif  BreakpointsForDimension2=dados.mach  BreakpointsForDimension3=dados.alpha  BreakpointsForDimension4=dados.cg  BreakpointsForDimension5=dados.phif  BreakpointsForDimension6=dados.mach  BreakpointsForDimension7=dados.alpha  BreakpointsForDimension8=dados.cg  Table=M.CMAD  ExtrapMethod=Clip  InternalRulePriority=Speed  RndMeth=Simplest  InputSameDT=on
      settings: InputPortMap=u0,u1,u2,u3
  CMQ : Lookup_n-D  NumberOfTableDimensions=4  BreakpointsForDimension1=dados.phif  BreakpointsForDimension2=dados.mach  BreakpointsForDimension3=dados.alpha  BreakpointsForDimension4=dados.cg  BreakpointsForDimension5=dados.phif  BreakpointsForDimension6=dados.mach  BreakpointsForDimension7=dados.alpha  BreakpointsForDimension8=dados.cg  Table=M.CMQ  ExtrapMethod=Clip  InternalRulePriority=Speed  RndMeth=Simplest  InputSameDT=on
      settings: InputPortMap=u0,u1,u2,u3
  Demux : Demux  Outputs=3
  Demux1 : Demux  Outputs=3
  Demux2 : Demux  Outputs=3
  Gain1 : Gain  Gain=c.R2D
  Gain2 : Gain  Gain=c.R2D
  Product{,1..3} (4 alike) : Product
  Terminator{1..6} (6 alike) : Terminator
  M : Outport  VectorParamsAs1DForOutWhenUnconnected=off
  wires:
  "Mach "/1 -> [mach]
  Gain2/1 -> [alfatotal]
  alfatotal/1 -> Gain2/1
  q/1 -> Product1/2
  qSd/1 -> Product/2
  Gain1/1 -> [phi]
  Add1/1 -> Product/1
  CMAD/1 -> Product3/1
  phi/1 -> Gain1/1
  CMQ/1 -> Product1/1
  alfaponto/1 -> Product3/2
  Add2/1 -> Product2/2
  d2V/1 -> Product2/1
  Product/1 -> M/1
  Product2/1 -> Add1/2
  CM/1 -> [CM]
  Product1/1 -> [CMQ]
  Product3/1 -> [CMAD]
  [CM] -> Add1/1
  [CMQ] -> Add2/1
  [CMAD] -> Add2/2
  cg/1 -> [CGa]
  [phi] -> CM/1
  [mach] -> CM/2
  [alfatotal] -> CM/3
  [phi] -> CMQ/1
  [mach] -> CMQ/2
  [alfatotal] -> CMQ/3
  [alfatotal] -> CMAD/3
  [mach] -> CMAD/2
  [phi] -> CMAD/1
  [CGa] -> Demux/1
  Demux/1 -> CM/4
  [CGa] -> Demux1/1
  Demux1/1 -> CMQ/4
  [CGa] -> Demux2/1
  Demux2/1 -> CMAD/4
  Demux2/2 -> Terminator1/1
  Demux2/3 -> Terminator2/1
  Demux/2 -> Terminator3/1
  Demux/3 -> Terminator4/1
  Demux1/2 -> Terminator5/1
  Demux1/3 -> Terminator6/1

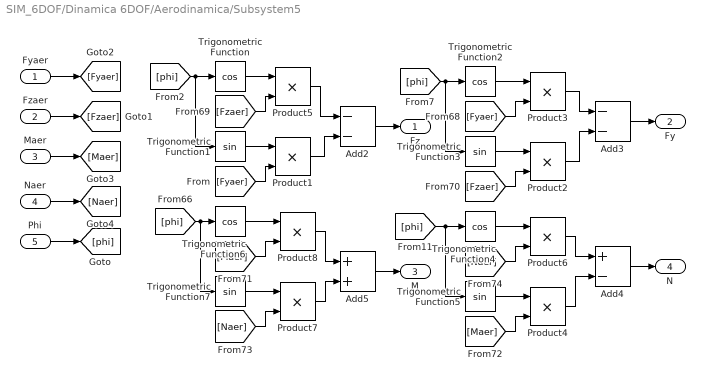
== system SIM_6DOF/Dinamica 6DOF/Aerodinamica/Subsystem5 ==
  Fyaer : Inport
  Fzaer : Inport  Port=2
  Maer : Inport  Port=3
  Naer : Inport  Port=4
  Phi : Inport  Port=5
  Add2 : Sum  Inputs=--
  Add3 : Sum  Inputs=--
  Add4 : Sum  Inputs=+-
  Add5 : Sum
  Product{1..8} (8 alike) : Product
  Trigonometric Function{,2,4,6} (4 alike) : Trigonometry  Operator=cos
  Trigonometric Function{1,3,5,7} (4 alike) : Trigonometry
  Fz : Outport  VectorParamsAs1DForOutWhenUnconnected=off
  Fy : Outport  Port=2  VectorParamsAs1DForOutWhenUnconnected=off
  M : Outport  Port=3  VectorParamsAs1DForOutWhenUnconnected=off
  N : Outport  Port=4  VectorParamsAs1DForOutWhenUnconnected=off
  wires:
  [phi] -> Trigonometric Function7/1, Trigonometric Function6/1
  Trigonometric Function6/1 -> Product8/1
  Trigonometric Function7/1 -> Product7/1
  Product8/1 -> Add5/1
  [phi] -> Trigonometric Function1/1, Trigonometric Function/1
  Trigonometric Function/1 -> Product5/1
  Trigonometric Function4/1 -> Product6/1
  [phi] -> Trigonometric Function5/1, Trigonometric Function4/1
  Trigonometric Function5/1 -> Product4/1
  [Naer] -> Product7/2
  [Maer] -> Product4/2
  [Fyaer] -> Product3/2
  [Fyaer] -> Product1/2
  [Maer] -> Product8/2
  Product7/1 -> Add5/2
  Trigonometric Function2/1 -> Product3/1
  Trigonometric Function3/1 -> Product2/1
  [phi] -> Trigonometric Function3/1, Trigonometric Function2/1
  [Fzaer] -> Product2/2
  [Naer] -> Product6/2
  Trigonometric Function1/1 -> Product1/1
  Phi/1 -> [phi]
  Fzaer/1 -> [Fzaer]
  Maer/1 -> [Maer]
  Naer/1 -> [Naer]
  Product1/1 -> Add2/2
  [Fzaer] -> Product5/2
  Product5/1 -> Add2/1
  Fyaer/1 -> [Fyaer]
  Product2/1 -> Add3/2
  Product3/1 -> Add3/1
  Product6/1 -> Add4/1
  Product4/1 -> Add4/2
  Add5/1 -> M/1
  Add2/1 -> Fz/1
  Add3/1 -> Fy/1
  Add4/1 -> N/1

== system SIM_6DOF/Dinamica 6DOF/Aerodinamica/Subsystem6 ==
  Forces : Inport
  CRM : Inport  Port=2
  CG : Inport  Port=3
  Moments CRM : Inport  Port=4
  3x3 Cross Product : sharedutil/3x3 Cross Product  aMode=aMode
      settings: SourceProductBaseCode=AE,PW,DR,MT,UV,VE
  Sum : Sum  Inputs=|+-  SaturateOnIntegerOverflow=on
  Sum1 : Sum  Inputs=++|  SaturateOnIntegerOverflow=on
  To Workspace : ToWorkspace  VariableName=Delta  SaveFormat=Timeseries  SampleTime=-1
  Moments CG : Outport  VectorParamsAs1DForOutWhenUnconnected=off
  wires:
  CRM/1 -> Sum/1
  CG/1 -> Sum/2
  Sum1/1 -> Moments CG/1
  Sum/1 -> 3x3 Cross Product/1, To Workspace/1
  Forces/1 -> 3x3 Cross Product/2
  Moments CRM/1 -> Sum1/1
  3x3 Cross Product/1 -> Sum1/2

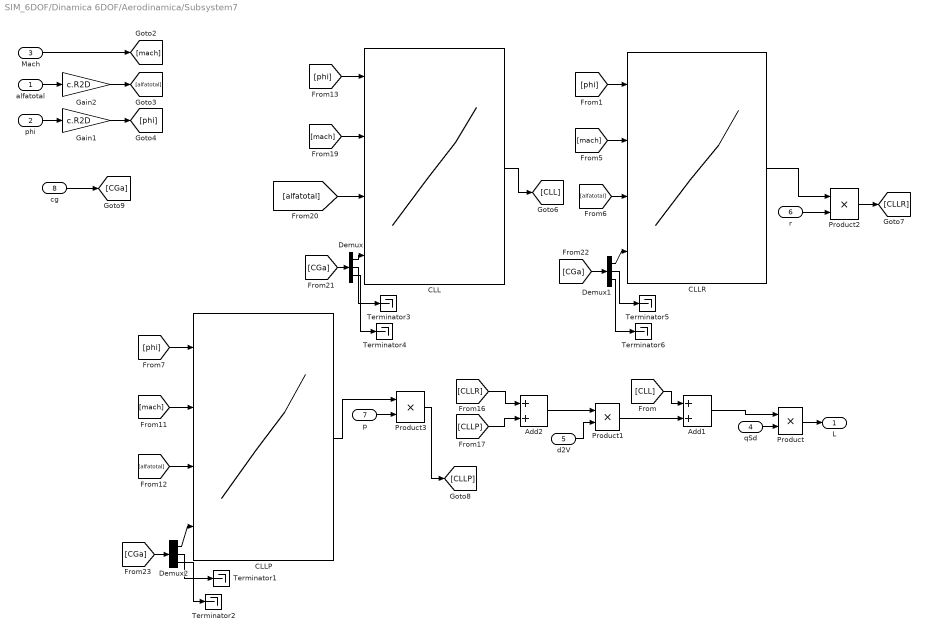
== system SIM_6DOF/Dinamica 6DOF/Aerodinamica/Subsystem7 ==
  alfatotal : Inport
  phi : Inport  Port=2
  "Mach " : Inport  Port=3
  qSd : Inport  Port=4
  d2V : Inport  Port=5
  r : Inport  Port=6
  p : Inport  Port=7
  cg : Inport  Port=8
  Add1 : Sum
  Add2 : Sum
  CLL : Lookup_n-D  NumberOfTableDimensions=4  BreakpointsForDimension1=dados.phif  BreakpointsForDimension2=dados.mach  BreakpointsForDimension3=dados.alpha  BreakpointsForDimension4=dados.cg  BreakpointsForDimension5=dados.phif  BreakpointsForDimension6=dados.mach  BreakpointsForDimension7=dados.alpha  BreakpointsForDimension8=dados.cg  Table=M.CLL  ExtrapMethod=Clip  InternalRulePriority=Speed  RndMeth=Simplest  InputSameDT=on
      settings: InputPortMap=u0,u1,u2,u3
  CLLP : Lookup_n-D  NumberOfTableDimensions=4  BreakpointsForDimension1=dados.phif  BreakpointsForDimension2=dados.mach  BreakpointsForDimension3=dados.alpha  BreakpointsForDimension4=dados.cg  BreakpointsForDimension5=dados.phif  BreakpointsForDimension6=dados.mach  BreakpointsForDimension7=dados.alpha  BreakpointsForDimension8=dados.cg  Table=M.CLLP  ExtrapMethod=Clip  InternalRulePriority=Speed  RndMeth=Simplest  InputSameDT=on
      settings: InputPortMap=u0,u1,u2,u3
  CLLR : Lookup_n-D  NumberOfTableDimensions=4  BreakpointsForDimension1=dados.phif  BreakpointsForDimension2=dados.mach  BreakpointsForDimension3=dados.alpha  BreakpointsForDimension4=dados.cg  BreakpointsForDimension5=dados.phif  BreakpointsForDimension6=dados.mach  BreakpointsForDimension7=dados.alpha  BreakpointsForDimension8=dados.cg  Table=M.CLLR  ExtrapMethod=Clip  InternalRulePriority=Speed  RndMeth=Simplest  InputSameDT=on
      settings: InputPortMap=u0,u1,u2,u3
  Demux : Demux  Outputs=3
  Demux1 : Demux  Outputs=3
  Demux2 : Demux  Outputs=3
  Gain1 : Gain  Gain=c.R2D
  Gain2 : Gain  Gain=c.R2D
  Product{,1..3} (4 alike) : Product
  Terminator{1..6} (6 alike) : Terminator
  L : Outport  VectorParamsAs1DForOutWhenUnconnected=off
  wires:
  p/1 -> Product3/2
  Add1/1 -> Product/1
  CLLP/1 -> Product3/1
  r/1 -> Product2/2
  Gain1/1 -> [phi]
  qSd/1 -> Product/2
  CLLR/1 -> Product2/1
  alfatotal/1 -> Gain2/1
  "Mach "/1 -> [mach]
  Gain2/1 -> [alfatotal]
  phi/1 -> Gain1/1
  Add2/1 -> Product1/1
  d2V/1 -> Product1/2
  Product1/1 -> Add1/2
  Product/1 -> L/1
  CLL/1 -> [CLL]
  [CLL] -> Add1/1
  Product2/1 -> [CLLR]
  Product3/1 -> [CLLP]
  [CLLR] -> Add2/1
  [CLLP] -> Add2/2
  cg/1 -> [CGa]
  [alfatotal] -> CLL/3
  [mach] -> CLL/2
  [phi] -> CLL/1
  [phi] -> CLLR/1
  [mach] -> CLLR/2
  [alfatotal] -> CLLR/3
  [phi] -> CLLP/1
  [mach] -> CLLP/2
  [alfatotal] -> CLLP/3
  [CGa] -> Demux/1
  Demux1/1 -> CLLR/4
  [CGa] -> Demux1/1
  Demux2/1 -> CLLP/4
  [CGa] -> Demux2/1
  Demux2/2 -> Terminator1/1
  Demux2/3 -> Terminator2/1
  Demux/2 -> Terminator3/1
  Demux/3 -> Terminator4/1
  Demux1/2 -> Terminator5/1
  Demux1/3 -> Terminator6/1
  Demux/1 -> CLL/4

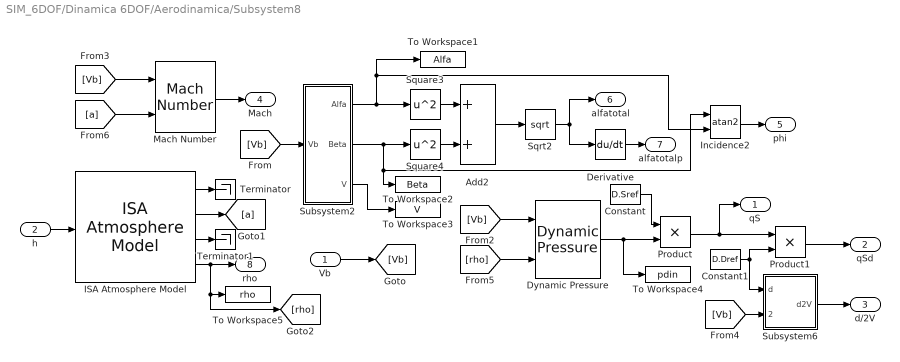
== system SIM_6DOF/Dinamica 6DOF/Aerodinamica/Subsystem8 ==
  Vb : Inport
  h : Inport  Port=2
  Add2 : Sum
  Constant : Constant  Value=D.Sref
  Constant1 : Constant  Value=D.Dref
  Derivative : Derivative
  Dynamic Pressure : aerolibasang/Dynamic Pressure
  ISA Atmosphere Model : aerolibatmos2/ISA Atmosphere Model  custom=off  g=9.80665  gamma=1.4  R=287.0531  L=0.0065  h_trop=11000  h_strat=20000  rho0=1.225  P0=101325  T0=288.15  h0=0
  Incidence2 : Trigonometry  Operator=atan2  OutputSignalType=real
  Mach Number : aerolibasang/Mach Number
      settings: SourceProductBaseCode=AE
  Product : Product
  Product1 : Product
  Sqrt2 : Sqrt  SaturateOnIntegerOverflow=on
  Square3 : Math  Operator=square  SignedPower=on  RndMeth=Zero  SaturateOnIntegerOverflow=on
  Square4 : Math  Operator=square  SignedPower=on  RndMeth=Zero  SaturateOnIntegerOverflow=on
  Subsystem2 : Subsystem
  Subsystem6 : Subsystem
  Terminator : Terminator
  Terminator1 : Terminator
  To Workspace1 : ToWorkspace  VariableName=Alfa  SaveFormat=Timeseries  SampleTime=-1
  To Workspace2 : ToWorkspace  VariableName=Beta  SaveFormat=Timeseries  SampleTime=-1
  To Workspace3 : ToWorkspace  VariableName=V  SaveFormat=Timeseries  SampleTime=-1
  To Workspace4 : ToWorkspace  VariableName=pdin  SaveFormat=Timeseries  SampleTime=-1
  To Workspace5 : ToWorkspace  VariableName=rho  SaveFormat=Timeseries  SampleTime=-1
  qS : Outport  VectorParamsAs1DForOutWhenUnconnected=off
  qSd : Outport  Port=2  VectorParamsAs1DForOutWhenUnconnected=off
  d/2V : Outport  Port=3  VectorParamsAs1DForOutWhenUnconnected=off
  Mach : Outport  Port=4  VectorParamsAs1DForOutWhenUnconnected=off
  phi : Outport  Port=5  VectorParamsAs1DForOutWhenUnconnected=off
  alfatotal : Outport  Port=6  VectorParamsAs1DForOutWhenUnconnected=off
  alfatotalp : Outport  Port=7  VectorParamsAs1DForOutWhenUnconnected=off
  rho : Outport  Port=8  VectorParamsAs1DForOutWhenUnconnected=off
  wires:
  h/1 -> ISA Atmosphere Model/1
  Constant/1 -> Product/1
  Dynamic Pressure/1 -> To Workspace4/1, Product/2
  ISA Atmosphere Model/4 -> [rho], To Workspace5/1, rho/1
  Constant1/1 -> Product1/2, Subsystem6/1(d)
  Product1/1 -> qSd/1
  Subsystem6/1(d2V) -> d/2V/1
  Product/1 -> Product1/1, qS/1
  Subsystem2/3(V) -> To Workspace3/1
  Mach Number/1 -> Mach/1
  [Vb] -> Subsystem2/1(Vb)
  [Vb] -> Dynamic Pressure/1
  [Vb] -> Mach Number/1
  [Vb] -> Subsystem6/2(Velocity)
  [rho] -> Dynamic Pressure/2
  [a] -> Mach Number/2
  ISA Atmosphere Model/2 -> [a]
  ISA Atmosphere Model/1 -> Terminator/1
  ISA Atmosphere Model/3 -> Terminator1/1
  Vb/1 -> [Vb]
  Derivative/1 -> alfatotalp/1
  Add2/1 -> Sqrt2/1
  Sqrt2/1 -> alfatotal/1, Derivative/1
  Incidence2/1 -> phi/1
  Square4/1 -> Add2/2
  Square3/1 -> Add2/1
  Subsystem2/2(Beta) -> To Workspace2/1, Incidence2/1, Square4/1
  Subsystem2/1(Alfa) -> Incidence2/2, To Workspace1/1, Square3/1

== system SIM_6DOF/Dinamica 6DOF/Aerodinamica/Subsystem8/Subsystem2 ==
  Vb : Inport
  Airspeed : Sqrt  AlgorithmType=Newton-Raphson  SaturateOnIntegerOverflow=on
  Incidence : Trigonometry  Operator=atan2
  Incidence1 : Trigonometry  Operator=atan2
  Subsystem : aerolibasang/Incidence, Sideslip, & Airspeed/Subsystem  SystemSampleTime=-1  VariantActivationTime=update diagram  Latency=0  AutoFrameSizeCalculation=off
      settings: SourceProductBaseCode=AE
  Subsystem1 : aerolibasang/Incidence, Sideslip, & Airspeed/Subsystem1  SystemSampleTime=-1  VariantActivationTime=update diagram  Latency=0  AutoFrameSizeCalculation=off
      settings: SourceProductBaseCode=AE
  dot : aerolibasang/Incidence, Sideslip, & Airspeed/dot  SystemSampleTime=-1  VariantActivationTime=update diagram  Latency=0  AutoFrameSizeCalculation=off
      settings: SourceProductBaseCode=AE
  Alfa : Outport  VectorParamsAs1DForOutWhenUnconnected=off
  Beta : Outport  Port=2  VectorParamsAs1DForOutWhenUnconnected=off
  V : Outport  Port=3  VectorParamsAs1DForOutWhenUnconnected=off
  wires:
  Subsystem1/1 -> Incidence1/1
  Incidence/1 -> Alfa/1
  Subsystem/1 -> Incidence/1
  dot/1 -> Airspeed/1
  Incidence1/1 -> Beta/1
  Subsystem/2 -> Incidence1/2, Incidence/2
  Vb/1 -> Subsystem1/1, dot/1, Subsystem/1
  Airspeed/1 -> V/1

== system SIM_6DOF/Dinamica 6DOF/Aerodinamica/Subsystem8/Subsystem6 ==
  d : Inport
  Velocity : Inport  Port=2
  Divide : Product  Inputs=*/
  d/(2V) : Gain  Gain=1/2  SaturateOnIntegerOverflow=on  OutDataTypeStr=Inherit: Same as input  ParamDataTypeStr=Inherit: Same as input
  dot : aerolibasang/Dynamic Pressure/dot  SystemSampleTime=-1  VariantActivationTime=update diagram  Latency=0  AutoFrameSizeCalculation=off
      settings: SourceProductBaseCode=AE
  vt : Sqrt  AlgorithmType=Newton-Raphson  SaturateOnIntegerOverflow=on
  d2V : Outport  InitialOutput=0  VectorParamsAs1DForOutWhenUnconnected=off
  wires:
  d/(2V)/1 -> d2V/1
  Velocity/1 -> dot/1
  Divide/1 -> d/(2V)/1
  dot/1 -> vt/1
  d/1 -> Divide/1
  vt/1 -> Divide/2
